simulink library "bcm"  (R2021b)
settings: Solver=VariableStepAuto  StartTime=0.0  StopTime=10.0  RelTol=1e-3
undefined symbols (not defined in the file or in its folder): KBCM_ShowUPT_cnt
libraries: simulink x33
(part 1 of 2)
settings Model: Creator=user  LastModifiedBy=FVT22063
settings SolverCC: AlgebraicLoopSolver=TrustRegion
settings DebuggingCC: SFMachineParentedDataDiag=warning

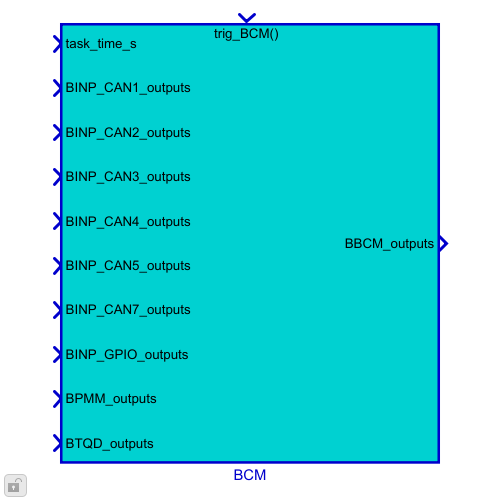
[thumbnail: Simulink's stored preview of the top-level diagram]
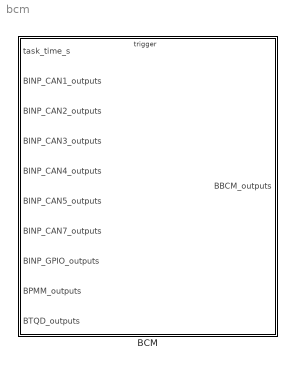
== system bcm ==
  BCM : Subsystem  TreatAsAtomicUnit=on
      settings: RTWSystemCode=Nonreusable function  RTWFcnNameOpts=Use subsystem name  RTWFileNameOpts=Use subsystem name

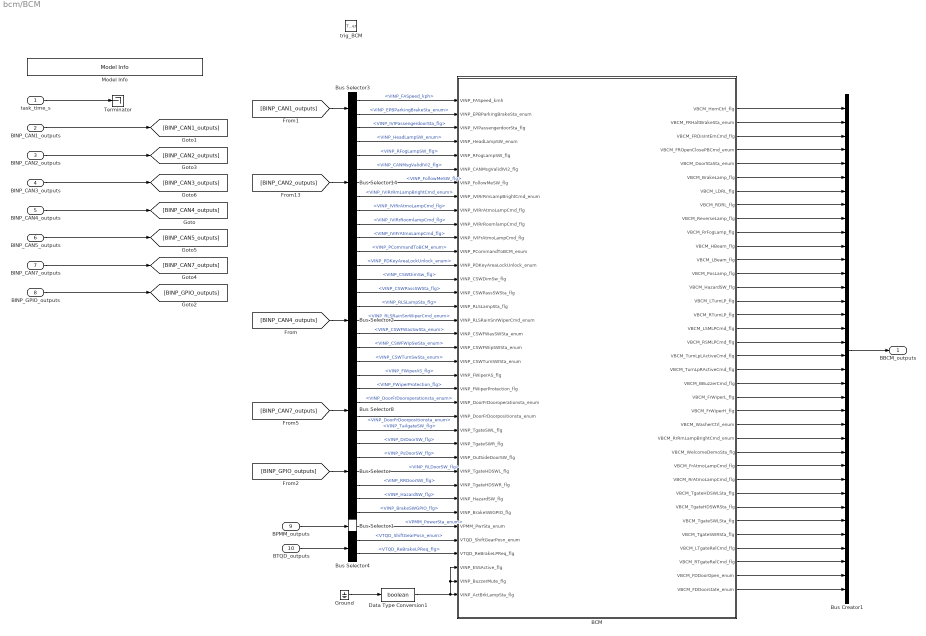
== system bcm/BCM ==
  task_time_s : Inport
  BINP_CAN1_outputs : Inport  Port=2  OutDataTypeStr=Bus: BINP_CAN1_outputs
  BINP_CAN2_outputs : Inport  Port=3  OutDataTypeStr=Bus: BINP_CAN2_outputs
  BINP_CAN3_outputs : Inport  Port=4  OutDataTypeStr=Bus: BINP_CAN3_outputs
  BINP_CAN4_outputs : Inport  Port=5  OutDataTypeStr=Bus: BINP_CAN4_outputs
  BINP_CAN5_outputs : Inport  Port=6  OutDataTypeStr=Bus: BINP_CAN5_outputs
  BINP_CAN7_outputs : Inport  Port=7  OutDataTypeStr=Bus: BINP_CAN7_outputs
  BINP_GPIO_outputs : Inport  Port=8  OutDataTypeStr=Bus: BINP_GPIO_outputs
  BPMM_outputs : Inport  Port=9  OutDataTypeStr=Bus: BPMM_outputs
  BTQD_outputs : Inport  Port=10  OutDataTypeStr=Bus: BTQD_outputs
  trig_BCM : TriggerPort  TriggerType=function-call  VariantControl=(inherit)
  BCM : Subsystem
  Bus Creator1 : BusCreator  Inputs=36  OutDataTypeStr=Bus: BBCM_outputs  NonVirtualBus=on
  Bus Selector : BusSelector  OutputSignals=VINP_TailgateSW_flg,VINP_DrDoorSW_flg,VINP_PsDoorSW_flg,VINP_RLDoorSW_flg,VINP_RRDoorSW_flg,VINP_HazardSW_flg,VINP_BrakeSWGPIO_flg
  Bus Selector1 : BusSelector  OutputSignals=VPMM_PowerSta_enum
  Bus Selector14 : BusSelector  OutputSignals=VINP_IVIPassengerdoorSta_flg,VINP_HeadLampSW_enum,VINP_RFogLampSW_flg,VINP_CANMsgValidIVI2_flg,VINP_FollowMeSW_flg,VINP_IVIRrRmLampBrightCmd_enum,VINP_IVIRrAtmoLampCmd_flg,VINP_IVIRrRoomlampCmd_flg,VINP_IVIFrAtmoLampCmd_flg
  Bus Selector2 : BusSelector  OutputSignals=VINP_PCommandToBCM_enum,VINP_PDKeyAreaLockUnlock_enum,VINP_CSWDimSw_flg,VINP_CSWPassSWSta_flg,VINP_RLSLampSta_flg,VINP_RLSRainSnrWiperCmd_enum,VINP_CSWFWasSwSta_enum,VINP_CSWFWipSwSta_enum,VINP_CSWTurnSwSta_enum,VINP_FWiperAS_flg,VINP_FWiperProtection_flg
  Bus Selector3 : BusSelector  OutputSignals=VINP_FASpeed_kph,VINP_EPBParkingBrakeSta_enum
  Bus Selector4 : BusSelector  OutputSignals=VTQD_ShiftGearPosn_enum,VTQD_ReBrakeLPReq_flg
  Bus Selector8 : BusSelector  OutputSignals=VINP_DoorFrDooroperationsta_enum,VINP_DoorFrDoorpositionsta_enum
  Data Type Conversion1 : DataTypeConversion  OutDataTypeStr=boolean
  Ground : Ground
  Model Info : simulink/Model-Wide Utilities/Model Info  Frame=on  DisplayStringWithTags=$Id: pmm.mdl 130 2021-02-08 12:40:01Z Shawn $  HorizontalTextAlignment=Center  LeftAlignmentValue=0.5
  Terminator : Terminator
  BBCM_outputs : Outport  OutDataTypeStr=Bus: BBCM_outputs  VectorParamsAs1DForOutWhenUnconnected=off
  wires:
  BPMM_outputs/1 -> Bus Selector1/1
  BINP_CAN4_outputs/1 -> [BINP_CAN4_outputs]
  BINP_CAN1_outputs/1 -> [BINP_CAN1_outputs]
  [BINP_CAN1_outputs] -> Bus Selector3/1
  BINP_GPIO_outputs/1 -> [BINP_GPIO_outputs]
  [BINP_GPIO_outputs] -> Bus Selector/1
  BINP_CAN2_outputs/1 -> [BINP_CAN2_outputs]
  BINP_CAN5_outputs/1 -> [BINP_CAN5_outputs]
  [BINP_CAN2_outputs] -> Bus Selector14/1
  BTQD_outputs/1 -> Bus Selector4/1
  [BINP_CAN4_outputs] -> Bus Selector2/1
  task_time_s/1 -> Terminator/1
  Bus Selector2/1 -> BCM/12(VINP_PCommandToBCM_enum)  "<VINP_PCommandToBCM_enum>"
  Bus Selector1/1 -> BCM/32(VPMM_PwrSta_enum)  "<VPMM_PowerSta_enum>"
  Bus Creator1/1 -> BBCM_outputs/1
  BINP_CAN3_outputs/1 -> [BINP_CAN3_outputs]
  Bus Selector3/1 -> BCM/1(VINP_FASpeed_kmh)  "<VINP_FASpeed_kph>"
  BCM/1(VBCM_HornCtrl_flg) -> Bus Creator1/1
  BCM/2(VBCM_FRHaltBrakeSta_enum) -> Bus Creator1/2
  BCM/3(VBCM_FRDisIntEmCmd_flg) -> Bus Creator1/3
  BCM/4(VBCM_FROpenClosePBCmd_enum) -> Bus Creator1/4
  BCM/5(VBCM_DoorStaSta_enum) -> Bus Creator1/5
  BCM/6(VBCM_BrakeLamp_flg) -> Bus Creator1/6
  BCM/7(VBCM_LDRL_flg) -> Bus Creator1/7
  BCM/8(VBCM_RDRL_flg) -> Bus Creator1/8
  BCM/9(VBCM_ReverseLamp_flg) -> Bus Creator1/9
  BCM/10(VBCM_RrFogLamp_flg) -> Bus Creator1/10
  BCM/11(VBCM_HBeam_flg) -> Bus Creator1/11
  BCM/12(VBCM_LBeam_flg) -> Bus Creator1/12
  BCM/13(VBCM_PosLamp_flg) -> Bus Creator1/13
  BCM/14(VBCM_HazardSW_flg) -> Bus Creator1/14
  BCM/15(VBCM_LTurnLP_flg) -> Bus Creator1/15
  BCM/16(VBCM_RTurnLP_flg) -> Bus Creator1/16
  BCM/17(VBCM_LSMLPCmd_flg) -> Bus Creator1/17
  BCM/18(VBCM_RSMLPCmd_flg) -> Bus Creator1/18
  BCM/19(VBCM_TurnLpLActiveCmd_flg) -> Bus Creator1/19
  BCM/20(VBCM_TurnLpRActiveCmd_flg) -> Bus Creator1/20
  BCM/21(VBCM_BBuzzerCmd_flg) -> Bus Creator1/21
  BCM/22(VBCM_FrWiperL_flg) -> Bus Creator1/22
  BCM/23(VBCM_FrWiperH_flg) -> Bus Creator1/23
  BCM/24(VBCM_WasherCtrl_enum) -> Bus Creator1/24
  BCM/25(VBCM_RrRmLampBrightCmd_enum) -> Bus Creator1/25
  BCM/26(VBCM_WelcomeDemoSta_flg) -> Bus Creator1/26
  BCM/27(VBCM_FrAtmoLampCmd_flg) -> Bus Creator1/27
  BCM/28(VBCM_RrAtmoLampCmd_flg) -> Bus Creator1/28
  BCM/29(VBCM_TgateHDSWLSta_flg) -> Bus Creator1/29
  BCM/30(VBCM_TgateHDSWRSta_flg) -> Bus Creator1/30
  BCM/31(VBCM_TgateSWLSta_flg) -> Bus Creator1/31
  BCM/32(VBCM_TgateSWRSta_flg) -> Bus Creator1/32
  BCM/33(VBCM_LTgateRelCmd_flg) -> Bus Creator1/33
  BCM/34(VBCM_RTgateRelCmd_flg) -> Bus Creator1/34
  BCM/35(VBCM_FDDoorOpen_enum) -> Bus Creator1/35
  BCM/36(VBCM_FDDoorstate_enum) -> Bus Creator1/36
  Bus Selector2/2 -> BCM/13(VINP_PDKeyAreaLockUnlock_enum)  "<VINP_PDKeyAreaLockUnlock_enum>"
  Bus Selector3/2 -> BCM/2(VINP_EPBParkingBrakeSta_enum)  "<VINP_EPBParkingBrakeSta_enum>"
  Bus Selector14/1 -> BCM/3(VINP_IVIPassengerdoorSta_flg)  "<VINP_IVIPassengerdoorSta_flg>"
  Bus Selector4/1 -> BCM/33(VTQD_ShiftGearPosn_enum)  "<VTQD_ShiftGearPosn_enum>"
  Bus Selector4/2 -> BCM/34(VTQD_ReBrakeLPReq_flg)  "<VTQD_ReBrakeLPReq_flg>"
  Bus Selector14/2 -> BCM/4(VINP_HeadLampSW_enum)  "<VINP_HeadLampSW_enum>"
  Bus Selector14/3 -> BCM/5(VINP_RFogLampSW_flg)  "<VINP_RFogLampSW_flg>"
  Bus Selector14/4 -> BCM/6(VINP_CANMsgValidIVI2_flg)  "<VINP_CANMsgValidIVI2_flg>"
  Bus Selector14/5 -> BCM/7(VINP_FollowMeSW_flg)  "<VINP_FollowMeSW_flg>"
  Bus Selector14/6 -> BCM/8(VINP_IVIRrRmLampBrightCmd_enum)  "<VINP_IVIRrRmLampBrightCmd_enum>"
  Bus Selector14/7 -> BCM/9(VINP_IVIRrAtmoLampCmd_flg)  "<VINP_IVIRrAtmoLampCmd_flg>"
  Bus Selector14/8 -> BCM/10(VINP_IVIRrRoomlampCmd_flg)  "<VINP_IVIRrRoomlampCmd_flg>"
  Bus Selector14/9 -> BCM/11(VINP_IVIFrAtmoLampCmd_flg)  "<VINP_IVIFrAtmoLampCmd_flg>"
  Bus Selector2/3 -> BCM/14(VINP_CSWDimSw_flg)  "<VINP_CSWDimSw_flg>"
  Bus Selector2/4 -> BCM/15(VINP_CSWPassSWSta_flg)  "<VINP_CSWPassSWSta_flg>"
  Bus Selector2/5 -> BCM/16(VINP_RLSLampSta_flg)  "<VINP_RLSLampSta_flg>"
  Bus Selector2/6 -> BCM/17(VINP_RLSRainSnrWiperCmd_enum)  "<VINP_RLSRainSnrWiperCmd_enum>"
  Bus Selector2/7 -> BCM/18(VINP_CSWFWasSWSta_enum)  "<VINP_CSWFWasSwSta_enum>"
  Bus Selector2/8 -> BCM/19(VINP_CSWFWipSWSta_enum)  "<VINP_CSWFWipSwSta_enum>"
  Bus Selector2/9 -> BCM/20(VINP_CSWTurnSWSta_enum)  "<VINP_CSWTurnSwSta_enum>"
  Data Type Conversion1/1 -> BCM/35(VINP_ESSActive_flg), BCM/36(VINP_BuzzerMute_flg), BCM/37(VINP_ActBrkLampSta_flg)
  Bus Selector2/10 -> BCM/21(VINP_FWiperAS_flg)  "<VINP_FWiperAS_flg>"
  Bus Selector2/11 -> BCM/22(VINP_FWiperProtection_flg)  "<VINP_FWiperProtection_flg>"
  BINP_CAN7_outputs/1 -> [BINP_CAN7_outputs]
  [BINP_CAN7_outputs] -> Bus Selector8/1
  Bus Selector8/1 -> BCM/23(VINP_DoorFrDooroperationsta_enum)  "<VINP_DoorFrDooroperationsta_enum>"
  Bus Selector8/2 -> BCM/24(VINP_DoorFrDoorpositionsta_enum)  "<VINP_DoorFrDoorpositionsta_enum>"
  Ground/1 -> Data Type Conversion1/1
  Bus Selector/3 -> BCM/27(VINP_OutSideDoorSW_flg)  "<VINP_PsDoorSW_flg>"
  Bus Selector/1 -> BCM/25(VINP_TgateSWL_flg)  "<VINP_TailgateSW_flg>"
  Bus Selector/4 -> BCM/28(VINP_TgateHDSWL_flg)  "<VINP_RLDoorSW_flg>"
  Bus Selector/5 -> BCM/29(VINP_TgateHDSWR_flg)  "<VINP_RRDoorSW_flg>"
  Bus Selector/7 -> BCM/31(VINP_BrakeSWGPIO_flg)  "<VINP_BrakeSWGPIO_flg>"
  Bus Selector/6 -> BCM/30(VINP_HazardSW_flg)  "<VINP_HazardSW_flg>"
  Bus Selector/2 -> BCM/26(VINP_TgateSWR_flg)  "<VINP_DrDoorSW_flg>"

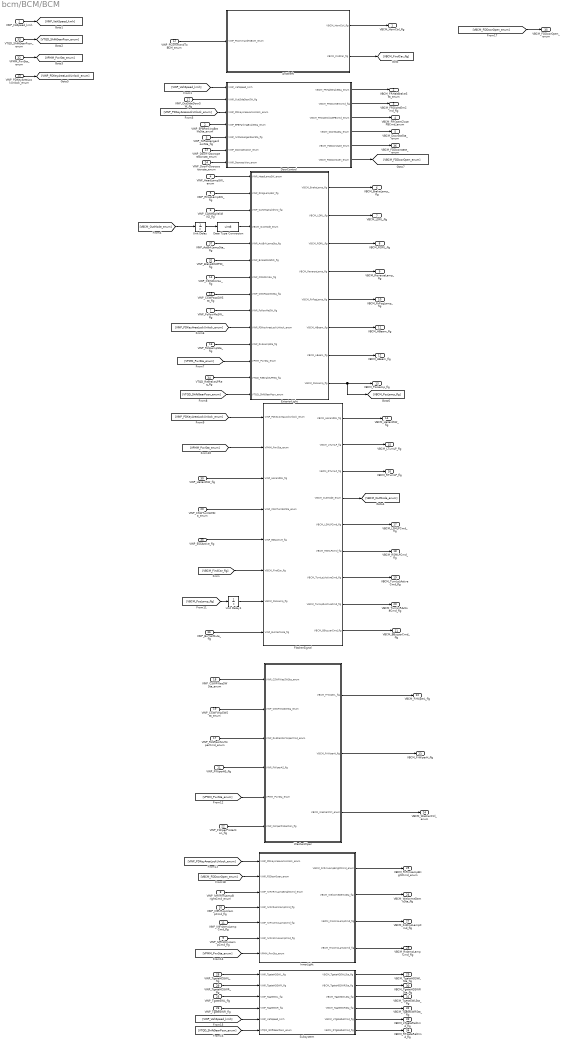
== system bcm/BCM/BCM ==
  VINP_FASpeed_kmh : Inport
  VINP_EPBParkingBrakeSta_enum : Inport  Port=2
  VINP_IVIPassengerdoorSta_flg : Inport  Port=3
  VINP_HeadLampSW_enum : Inport  Port=4
  VINP_RFogLampSW_flg : Inport  Port=5
  VINP_CANMsgValidIVI2_flg : Inport  Port=6
  VINP_FollowMeSW_flg : Inport  Port=7
  VINP_IVIRrRmLampBrightCmd_enum : Inport  Port=8
  VINP_IVIRrAtmoLampCmd_flg : Inport  Port=9
  VINP_IVIRrRoomlampCmd_flg : Inport  Port=10
  VINP_IVIFrAtmoLampCmd_flg : Inport  Port=11
  VINP_PCommandToBCM_enum : Inport  Port=12
  VINP_PDKeyAreaLockUnlock_enum : Inport  Port=13
  VINP_CSWDimSw_flg : Inport  Port=14
  VINP_CSWPassSWSta_flg : Inport  Port=15
  VINP_RLSLampSta_flg : Inport  Port=16
  VINP_RLSRainSnrWiperCmd_enum : Inport  Port=17
  VINP_CSWFWasSWSta_enum : Inport  Port=18
  VINP_CSWFWipSWSta_enum : Inport  Port=19
  VINP_CSWTurnSWSta_enum : Inport  Port=20
  VINP_FWiperAS_flg : Inport  Port=21
  VINP_FWiperProtection_flg : Inport  Port=22
  VINP_DoorFrDooroperationsta_enum : Inport  Port=23
  VINP_DoorFrDoorpositionsta_enum : Inport  Port=24
  VINP_TgateSWL_flg : Inport  Port=25
  VINP_TgateSWR_flg : Inport  Port=26
  VINP_OutSideDoorSW_flg : Inport  Port=27
  VINP_TgateHDSWL_flg : Inport  Port=28
  VINP_TgateHDSWR_flg : Inport  Port=29
  VINP_HazardSW_flg : Inport  Port=30
  VINP_BrakeSWGPIO_flg : Inport  Port=31
  VPMM_PwrSta_enum : Inport  Port=32
  VTQD_ShiftGearPosn_enum : Inport  Port=33
  VTQD_ReBrakeLPReq_flg : Inport  Port=34
  VINP_ESSActive_flg : Inport  Port=35
  VINP_BuzzerMute_flg : Inport  Port=36
  VINP_ActBrkLampSta_flg : Inport  Port=37
  Antitheft : Subsystem
  Data Type Conversion : DataTypeConversion  OutDataTypeStr=uint8
  DoorControl : Subsystem
  ExteriorLight : Subsystem
  FlasherSignal : Subsystem
  InnerLight : Subsystem
  Subsystem : Subsystem
  Unit Delay : UnitDelay  SampleTime=-1  HasFrameUpgradeWarning=on
  Unit Delay1 : UnitDelay  SampleTime=-1  HasFrameUpgradeWarning=on
  WasherWiper : Subsystem
  VBCM_HornCtrl_flg : Outport
  VBCM_FRHaltBrakeSta_enum : Outport  Port=2
  VBCM_FRDisIntEmCmd_flg : Outport  Port=3
  VBCM_FROpenClosePBCmd_enum : Outport  Port=4
  VBCM_DoorStaSta_enum : Outport  Port=5
  VBCM_BrakeLamp_flg : Outport  Port=6
  VBCM_LDRL_flg : Outport  Port=7
  VBCM_RDRL_flg : Outport  Port=8
  VBCM_ReverseLamp_flg : Outport  Port=9
  VBCM_RrFogLamp_flg : Outport  Port=10
  VBCM_HBeam_flg : Outport  Port=11
  VBCM_LBeam_flg : Outport  Port=12
  VBCM_PosLamp_flg : Outport  Port=13
  VBCM_HazardSW_flg : Outport  Port=14
  VBCM_LTurnLP_flg : Outport  Port=15
  VBCM_RTurnLP_flg : Outport  Port=16
  VBCM_LSMLPCmd_flg : Outport  Port=17
  VBCM_RSMLPCmd_flg : Outport  Port=18
  VBCM_TurnLpLActiveCmd_flg : Outport  Port=19
  VBCM_TurnLpRActiveCmd_flg : Outport  Port=20
  VBCM_BBuzzerCmd_flg : Outport  Port=21
  VBCM_FrWiperL_flg : Outport  Port=22
  VBCM_FrWiperH_flg : Outport  Port=23
  VBCM_WasherCtrl_enum : Outport  Port=24
  VBCM_RrRmLampBrightCmd_enum : Outport  Port=25
  VBCM_WelcomeDemoSta_flg : Outport  Port=26
  VBCM_FrAtmoLampCmd_flg : Outport  Port=27
  VBCM_RrAtmoLampCmd_flg : Outport  Port=28
  VBCM_TgateHDSWLSta_flg : Outport  Port=29
  VBCM_TgateHDSWRSta_flg : Outport  Port=30
  VBCM_TgateSWLSta_flg : Outport  Port=31
  VBCM_TgateSWRSta_flg : Outport  Port=32
  VBCM_LTgateRelCmd_flg : Outport  Port=33
  VBCM_RTgateRelCmd_flg : Outport  Port=34
  VBCM_FDDoorOpen_enum : Outport  Port=35
  VBCM_FDDoorstate_enum : Outport  Port=36
  wires:
  FlasherSignal/6(VBCM_RSMLPCmd_flg) -> VBCM_RSMLPCmd_flg/1
  VINP_ActBrkLampSta_flg/1 -> ExteriorLight/5(VINP_ActBrkLampSta_flg)
  VINP_IVIRrAtmoLampCmd_flg/1 -> InnerLight/6(VINP_IVIRrAtmoLampCmd_flg)
  VINP_TgateSWR_flg/1 -> Subsystem/4(VINP_TgateSWR_flg)
  VINP_TgateHDSWR_flg/1 -> Subsystem/2(VINP_TgateHDSWR_flg)
  VINP_ESSActive_flg/1 -> FlasherSignal/5(VINP_ESSActive_flg)
  VINP_TgateHDSWL_flg/1 -> Subsystem/1(VINP_TgateHDSWL_flg)
  FlasherSignal/5(VBCM_LSMLPCmd_flg) -> VBCM_LSMLPCmd_flg/1
  VINP_IVIRrRoomlampCmd_flg/1 -> InnerLight/4(VINP_IVIRrRoomlampCmd_flg)
  VINP_IVIFrAtmoLampCmd_flg/1 -> InnerLight/5(VINP_IVIFrAtmoLampCmd_flg)
  FlasherSignal/4(VBCM_OutMode_enum) -> [VBCM_OutMode_enum]
  VINP_IVIRrRmLampBrightCmd_enum/1 -> InnerLight/3(VINP_IVIRrRmLampBrightCmd_enum)
  [VINP_VehSpeed_kmh] -> Subsystem/5(VINP_VehSpeed_kmh)
  VINP_HeadLampSW_enum/1 -> ExteriorLight/1(VINP_HeadLampSW_enum)
  [VINP_PDKeyAreaLockUnlock_enum] -> FlasherSignal/1(VINP_PDKeyAreaLockUnlock_enum)
  VINP_FWiperAS_flg/1 -> WasherWiper/4(VINP_FWiperAS_flg)
  [VPMM_PwrSta_enum] -> ExteriorLight/12(VPMM_PwrSta_enum)
  Unit Delay1/1 -> FlasherSignal/7(VBCM_PosLamp_flg)
  [VINP_PDKeyAreaLockUnlock_enum] -> DoorControl/3(VINP_PDKeyAreaLockUnlock_enum)
  DoorControl/1(VBCM_FRHaltBrakeSta_enum) -> VBCM_FRHaltBrakeSta_enum/1
  VINP_RLSRainSnrWiperCmd_enum/1 -> WasherWiper/3(VINP_RLSRainSnrWiperCmd_enum)
  VINP_CSWFWipSWSta_enum/1 -> WasherWiper/2(VINP_CSWFWipSWSta_enum)
  [VBCM_PosLamp_flg] -> Unit Delay1/1
  VINP_BuzzerMute_flg/1 -> FlasherSignal/8(VINP_BuzzerMute_flg)
  VINP_FWiperProtection_flg/1 -> WasherWiper/6(VINP_FWiperProtection_flg)
  [VINP_PDKeyAreaLockUnlock_enum] -> InnerLight/1(VINP_PDKeyAreaLockUnlock_enum)
  VINP_CSWFWasSWSta_enum/1 -> WasherWiper/1(VINP_CSWFWasSWSta_enum)
  VINP_BrakeSWGPIO_flg/1 -> ExteriorLight/6(VINP_BrakeSWGPIO_flg)
  ExteriorLight/4(VBCM_ReverseLamp_flg) -> VBCM_ReverseLamp_flg/1
  [VPMM_PwrSta_enum] -> WasherWiper/5(VPMM_PwrSta_enum)
  VINP_CSWTurnSWSta_enum/1 -> FlasherSignal/4(VINP_CSWTurnSWSta_enum)
  [VINP_PDKeyAreaLockUnlock_enum] -> ExteriorLight/10(VINP_PDKeyAreaLockUnlock_enum)
  VINP_HazardSW_flg/1 -> FlasherSignal/3(VINP_HazardSW_flg)
  VINP_CANMsgValidIVI2_flg/1 -> ExteriorLight/3(VINP_CANMsgValidIVI2_flg)
  VINP_CSWDimSw_flg/1 -> ExteriorLight/7(VINP_CSWDimSw_flg)
  [VTQD_ShiftGearPosn_enum] -> ExteriorLight/14(VTQD_ShiftGearPosn_enum)
  ExteriorLight/2(VBCM_LDRL_flg) -> VBCM_LDRL_flg/1
  VINP_RLSLampSta_flg/1 -> ExteriorLight/11(VINP_RLSLampSta_flg)
  VINP_CSWPassSWSta_flg/1 -> ExteriorLight/8(VINP_CSWPassSWSta_flg)
  VINP_PDKeyAreaLockUnlock_enum/1 -> [VINP_PDKeyAreaLockUnlock_enum]
  VINP_RFogLampSW_flg/1 -> ExteriorLight/2(VINP_RFogLampSW_flg)
  VINP_EPBParkingBrakeSta_enum/1 -> DoorControl/4(VINP_EPBParkingBrakeSta_enum)
  VINP_FASpeed_kmh/1 -> [VINP_VehSpeed_kmh]
  DoorControl/4(VBCM_DoorStaSta_enum) -> VBCM_DoorStaSta_enum/1
  Unit Delay/1 -> Data Type Conversion/1
  Antitheft/2(VBCM_FindCar_flg) -> [VBCM_FindCar_flg]
  [VBCM_FindCar_flg] -> FlasherSignal/6(VBCM_FindCar_flg)
  Antitheft/1(VBCM_HornCtrl_flg) -> VBCM_HornCtrl_flg/1
  InnerLight/4(VBCM_RrAtmoLampCmd_flg) -> VBCM_RrAtmoLampCmd_flg/1
  FlasherSignal/9(VBCM_BBuzzerCmd_flg) -> VBCM_BBuzzerCmd_flg/1
  InnerLight/2(VBCM_WelcomeDemoSta_flg) -> VBCM_WelcomeDemoSta_flg/1
  [VBCM_OutMode_enum] -> Unit Delay/1
  ExteriorLight/3(VBCM_RDRL_flg) -> VBCM_RDRL_flg/1
  FlasherSignal/3(VBCM_RTurnLP_flg) -> VBCM_RTurnLP_flg/1
  WasherWiper/1(VBCM_FrWiperL_flg) -> VBCM_FrWiperL_flg/1
  VINP_PCommandToBCM_enum/1 -> Antitheft/1(VINP_PCommandToBCM_enum)
  VINP_TgateSWL_flg/1 -> Subsystem/3(VINP_TgateSWL_flg)
  ExteriorLight/5(VBCM_RrFogLamp_flg) -> VBCM_RrFogLamp_flg/1
  InnerLight/3(VBCM_FrAtmoLampCmd_flg) -> VBCM_FrAtmoLampCmd_flg/1
  InnerLight/1(VBCM_RrRmLampBrightCmd_enum) -> VBCM_RrRmLampBrightCmd_enum/1
  DoorControl/2(VBCM_FRDisIntEmCmd_flg) -> VBCM_FRDisIntEmCmd_flg/1
  VPMM_PwrSta_enum/1 -> [VPMM_PwrSta_enum]
  VINP_FollowMeSW_flg/1 -> ExteriorLight/9(VINP_FollowMeSW_flg)
  VINP_IVIPassengerdoorSta_flg/1 -> DoorControl/5(VINP_IVIPassengerdoorSta_flg)
  WasherWiper/2(VBCM_FrWiperH_flg) -> VBCM_FrWiperH_flg/1
  ExteriorLight/8(VBCM_PosLamp_flg) -> [VBCM_PosLamp_flg], VBCM_PosLamp_flg/1
  [VBCM_FDDoorOpen_enum] -> VBCM_FDDoorOpen_enum/1
  DoorControl/6(VBCM_FDDoorOpen_enum) -> [VBCM_FDDoorOpen_enum]
  Subsystem/6(VBCM_RTgateRelCmd_flg) -> VBCM_RTgateRelCmd_flg/1
  Subsystem/1(VBCM_TgateHDSWLSta_flg) -> VBCM_TgateHDSWLSta_flg/1
  VINP_OutSideDoorSW_flg/1 -> DoorControl/2(VINP_OutSideDoorSW_flg)
  Subsystem/2(VBCM_TgateHDSWRSta_flg) -> VBCM_TgateHDSWRSta_flg/1
  [VPMM_PwrSta_enum] -> FlasherSignal/2(VPMM_PwrSta_enum)
  VTQD_ReBrakeLPReq_flg/1 -> ExteriorLight/13(VTQD_ReBrakeLPReq_flg)
  VTQD_ShiftGearPosn_enum/1 -> [VTQD_ShiftGearPosn_enum]
  Subsystem/4(VBCM_TgateSWRSta_flg) -> VBCM_TgateSWRSta_flg/1
  WasherWiper/3(VBCM_WasherCtrl_enum) -> VBCM_WasherCtrl_enum/1
  DoorControl/3(VBCM_FROpenClosePBCmd_enum) -> VBCM_FROpenClosePBCmd_enum/1
  Subsystem/5(VBCM_LTgateRelCmd_flg) -> VBCM_LTgateRelCmd_flg/1
  [VBCM_FDDoorOpen_enum] -> InnerLight/2(VINP_FDDoorOpen_enum)
  FlasherSignal/8(VBCM_TurnLpRActiveCmd_flg) -> VBCM_TurnLpRActiveCmd_flg/1
  ExteriorLight/1(VBCM_BrakeLamp_flg) -> VBCM_BrakeLamp_flg/1
  [VPMM_PwrSta_enum] -> InnerLight/7(VPMM_PwrSta_enum)
  Subsystem/3(VBCM_TgateSWLSta_flg) -> VBCM_TgateSWLSta_flg/1
  FlasherSignal/7(VBCM_TurnLpLActiveCmd_flg) -> VBCM_TurnLpLActiveCmd_flg/1
  [VTQD_ShiftGearPosn_enum] -> Subsystem/6(VTQD_ShiftGearPosn_enum)
  ExteriorLight/6(VBCM_HBeam_flg) -> VBCM_HBeam_flg/1
  [VINP_VehSpeed_kmh] -> DoorControl/1(VINP_VehSpeed_kmh)
  FlasherSignal/2(VBCM_LTurnLP_flg) -> VBCM_LTurnLP_flg/1
  FlasherSignal/1(VBCM_HazardSW_flg) -> VBCM_HazardSW_flg/1
  ExteriorLight/7(VBCM_LBeam_flg) -> VBCM_LBeam_flg/1
  VINP_DoorFrDooroperationsta_enum/1 -> DoorControl/6(VINP_Dooroperation_enum)
  VINP_DoorFrDoorpositionsta_enum/1 -> DoorControl/7(VINP_Doorposition_enum)
  DoorControl/5(VBCM_FDDoorstate_enum) -> VBCM_FDDoorstate_enum/1
  Data Type Conversion/1 -> ExteriorLight/4(VBCM_OutMode_enum)

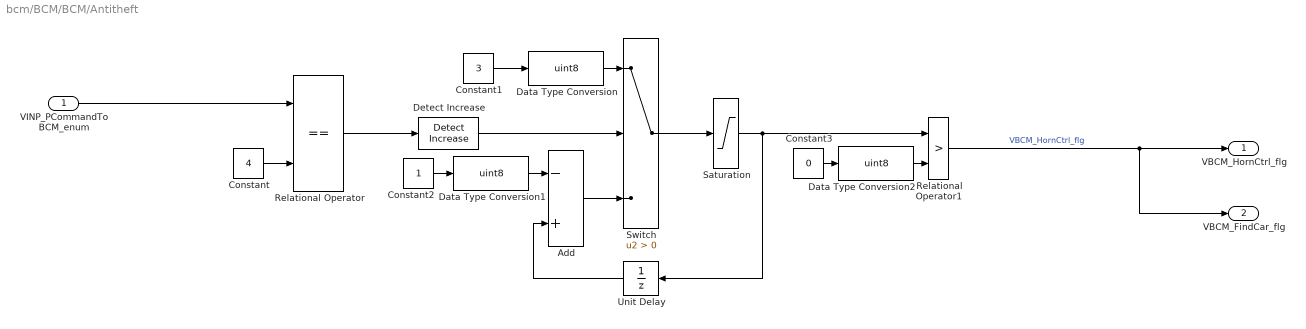
== system bcm/BCM/BCM/Antitheft ==
  VINP_PCommandToBCM_enum : Inport
  Add : Sum  Inputs=-+
  Constant : Constant  Value=4
  Constant1 : Constant  Value=3
  Constant2 : Constant
  Constant3 : Constant  Value=0
  Data Type Conversion : DataTypeConversion  OutDataTypeStr=uint8
  Data Type Conversion1 : DataTypeConversion  OutDataTypeStr=uint8
  Data Type Conversion2 : DataTypeConversion  OutDataTypeStr=uint8
  Detect Increase : simulink/Logic and Bit Operations/Detect Increase  vinit=0.0  OutDataTypeStr=boolean
  Relational Operator : RelationalOperator  Operator===  OutDataTypeStr=boolean  RndMeth=Simplest
  Relational Operator1 : RelationalOperator  Operator=>  OutDataTypeStr=boolean  RndMeth=Simplest
  Saturation : Saturate  UpperLimit=3  LowerLimit=0
  Switch : Switch  Criteria=u2 > Threshold
  Unit Delay : UnitDelay  SampleTime=-1  HasFrameUpgradeWarning=on
  VBCM_HornCtrl_flg : Outport
  VBCM_FindCar_flg : Outport  Port=2
  wires:
  Relational Operator1/1 -> VBCM_FindCar_flg/1, VBCM_HornCtrl_flg/1  "VBCM_HornCtrl_flg"
  Constant2/1 -> Data Type Conversion1/1
  Data Type Conversion1/1 -> Add/1
  Saturation/1 -> Unit Delay/1, Relational Operator1/1
  Detect Increase/1 -> Switch/2
  VINP_PCommandToBCM_enum/1 -> Relational Operator/1
  Data Type Conversion/1 -> Switch/1
  Switch/1 -> Saturation/1
  Constant1/1 -> Data Type Conversion/1
  Data Type Conversion2/1 -> Relational Operator1/2
  Constant/1 -> Relational Operator/2
  Constant3/1 -> Data Type Conversion2/1
  Relational Operator/1 -> Detect Increase/1
  Unit Delay/1 -> Add/2
  Add/1 -> Switch/3

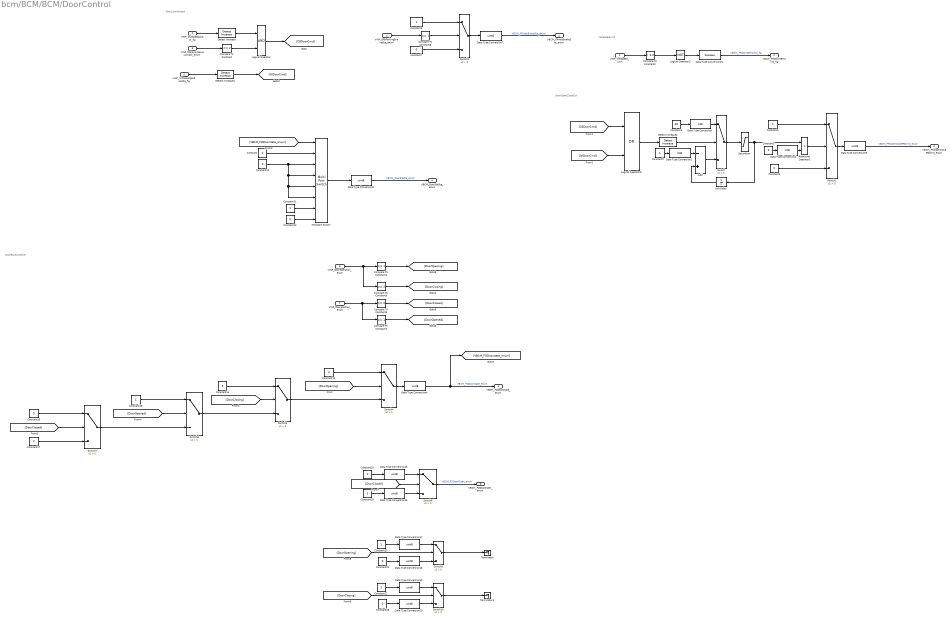
== system bcm/BCM/BCM/DoorControl ==
  note: DoorECUtoVehcle
  note: VehSpeedLimit
  note: DoorOpenCloseCtrl
  note: DoorControlInput
  VINP_VehSpeed_kmh : Inport
  VINP_OutSideDoorSW_flg : Inport  Port=2
  VINP_PDKeyAreaLockUnlock_enum : Inport  Port=3
  VINP_EPBParkingBrakeSta_enum : Inport  Port=4
  VINP_IVIPassengerdoorSta_flg : Inport  Port=5
  VINP_Dooroperation_enum : Inport  Port=6
  VINP_Doorposition_enum : Inport  Port=7
  Add : Sum  Inputs=-+
  Compare To Constant : simulink/Logic and Bit Operations/Compare To Constant  relop===  const=2  OutDataTypeStr=boolean
  Compare To Constant2 : simulink/Logic and Bit Operations/Compare To Constant  relop=>  const=3.0  OutDataTypeStr=boolean
  Compare To Constant3 : simulink/Logic and Bit Operations/Compare To Constant  relop===  const=1  OutDataTypeStr=boolean
  Compare To Constant4 : simulink/Logic and Bit Operations/Compare To Constant  relop===  const=1  OutDataTypeStr=boolean
  Compare To Constant5 : simulink/Logic and Bit Operations/Compare To Constant  relop===  const=2  OutDataTypeStr=boolean
  Compare To Constant6 : simulink/Logic and Bit Operations/Compare To Constant  relop===  const=0  OutDataTypeStr=boolean
  Compare To Constant7 : simulink/Logic and Bit Operations/Compare To Constant  relop===  const=1  OutDataTypeStr=boolean
  Constant : Constant  Value=2
  Constant1 : Constant  Value=30
  Constant{3,5,7,10,16,18,21,23} (8 alike) : Constant  Value=0
  Constant{2,4,6,11,15,19..20,22} (8 alike) : Constant
  Constant12 : Constant  Value=2
  Constant13 : Constant  Value=4
  Constant14 : Constant  Value=5
  Constant17 : Constant  Value=2
  Data Type Conversion : DataTypeConversion  OutDataTypeStr=int8
  Data Type Conversion1 : DataTypeConversion  OutDataTypeStr=int8
  Data Type Conversion{4..5,7,9,15..20} (10 alike) : DataTypeConversion  OutDataTypeStr=uint8
  Data Type Conversion2 : DataTypeConversion  OutDataTypeStr=int8
  Data Type Conversion21 : DataTypeConversion  OutDataTypeStr=boolean
  Detect Increase : simulink/Logic and Bit Operations/Detect Increase  vinit=0.0  OutDataTypeStr=boolean
  Detect Increase1 : simulink/Logic and Bit Operations/Detect Increase  vinit=0.0  OutDataTypeStr=boolean
  Detect Increase2 : simulink/Logic and Bit Operations/Detect Increase  vinit=0.0  OutDataTypeStr=boolean
  Logical Operator : Logic  AllPortsSameDT=off  OutDataTypeStr=boolean
  Logical Operator2 : Logic  Operator=NOT  AllPortsSameDT=off  OutDataTypeStr=boolean
  Logical Operator3 : Logic  Operator=OR  AllPortsSameDT=off  OutDataTypeStr=boolean
  Multiport Switch : MultiPortSwitch  DataPortOrder=Zero-based contiguous  Inputs=7  DiagnosticForDefault=None  zeroidx=on
  Relational Operator1 : RelationalOperator  Operator=>  OutDataTypeStr=boolean  RndMeth=Simplest
  Saturation : Saturate  UpperLimit=30  LowerLimit=0
  Switch{,1..2,4..10} (10 alike) : Switch  Criteria=u2 > Threshold
  Terminator : Terminator
  Terminator1 : Terminator
  Unit Delay : UnitDelay  SampleTime=-1  HasFrameUpgradeWarning=on
  VBCM_FRHaltBrakeSta_enum : Outport
  VBCM_FRDisIntEmCmd_flg : Outport  Port=2
  VBCM_FROpenClosePBCmd_enum : Outport  Port=3
  VBCM_DoorStaSta_enum : Outport  Port=4
  VBCM_FDDoorstate_enum : Outport  Port=5
  VBCM_FDDoorOpen_enum : Outport  Port=6
  wires:
  VINP_OutSideDoorSW_flg/1 -> Detect Increase/1
  VINP_PDKeyAreaLockUnlock_enum/1 -> Compare To Constant/1
  Detect Increase/1 -> Logical Operator/1
  Compare To Constant/1 -> Logical Operator/2
  Logical Operator/1 -> [OSDoorCmd]
  VINP_IVIPassengerdoorSta_flg/1 -> Detect Increase1/1
  Detect Increase1/1 -> [IVIDoorCmd]
  VINP_VehSpeed_kmh/1 -> Compare To Constant2/1
  Compare To Constant2/1 -> Logical Operator2/1
  Logical Operator2/1 -> Data Type Conversion21/1
  [OSDoorCmd] -> Logical Operator3/1
  [IVIDoorCmd] -> Logical Operator3/2
  Add/1 -> Switch/3
  Logical Operator3/1 -> Detect Increase2/1
  Unit Delay/1 -> Add/2
  Constant3/1 -> Data Type Conversion2/1
  Data Type Conversion2/1 -> Relational Operator1/2
  Detect Increase2/1 -> Switch/2
  Constant2/1 -> Data Type Conversion1/1
  Saturation/1 -> Unit Delay/1, Relational Operator1/1
  Data Type Conversion1/1 -> Add/1
  Switch/1 -> Saturation/1
  Constant1/1 -> Data Type Conversion/1
  Data Type Conversion/1 -> Switch/1
  Switch1/1 -> Data Type Conversion5/1
  Relational Operator1/1 -> Switch1/2
  Constant4/1 -> Switch1/1
  VINP_EPBParkingBrakeSta_enum/1 -> Compare To Constant3/1
  Compare To Constant3/1 -> Switch2/2
  Switch2/1 -> Data Type Conversion7/1
  Constant6/1 -> Switch2/1
  Constant7/1 -> Switch2/3
  Constant/1 -> Multiport Switch/2
  Multiport Switch/1 -> Data Type Conversion9/1
  Constant10/1 -> Multiport Switch/6, Multiport Switch/5, Multiport Switch/4, Multiport Switch/3
  Constant11/1 -> Multiport Switch/7
  Data Type Conversion9/1 -> VBCM_DoorStaSta_enum/1  "VBCM_DoorStaSta_enum"
  Constant12/1 -> Multiport Switch/8
  VINP_Dooroperation_enum/1 -> Compare To Constant5/1, Compare To Constant4/1
  Compare To Constant4/1 -> [DoorOpening]
  Compare To Constant5/1 -> [DoorClosing]
  VINP_Doorposition_enum/1 -> Compare To Constant7/1, Compare To Constant6/1
  Compare To Constant6/1 -> [DoorClosed]
  Compare To Constant7/1 -> [DoorOpened]
  [DoorOpening] -> Switch4/2
  Constant13/1 -> Switch4/1
  Switch5/1 -> Switch4/3
  [DoorClosing] -> Switch5/2
  Constant14/1 -> Switch5/1
  Switch6/1 -> Switch5/3
  [DoorOpened] -> Switch6/2
  Constant15/1 -> Switch6/1
  Constant16/1 -> Switch7/1
  [DoorClosed] -> Switch7/2
  Switch7/1 -> Switch6/3
  Constant17/1 -> Switch7/3
  Switch4/1 -> Data Type Conversion4/1
  [VBCM_FDDoorstate_enum] -> Multiport Switch/1
  [DoorClosed] -> Switch8/2
  Constant18/1 -> Data Type Conversion15/1
  Data Type Conversion15/1 -> Switch8/1
  Constant19/1 -> Data Type Conversion16/1
  Data Type Conversion16/1 -> Switch8/3
  Switch8/1 -> VBCM_FDDoorOpen_enum/1  "VBCM_FDDoorOpen_enum"
  [DoorOpening] -> Switch9/2
  Data Type Conversion17/1 -> Switch9/1
  Constant20/1 -> Data Type Conversion17/1
  Data Type Conversion18/1 -> Switch9/3
  Constant21/1 -> Data Type Conversion18/1
  Switch9/1 -> Terminator/1
  Switch10/1 -> Terminator1/1
  Constant23/1 -> Data Type Conversion20/1
  Data Type Conversion20/1 -> Switch10/3
  Constant22/1 -> Data Type Conversion19/1
  Data Type Conversion19/1 -> Switch10/1
  [DoorClosing] -> Switch10/2
  Data Type Conversion21/1 -> VBCM_FRDisIntEmCmd_flg/1  "VBCM_FRDisIntEmCmd_flg"
  Data Type Conversion7/1 -> VBCM_FRHaltBrakeSta_enum/1  "VBCM_FRHaltBrakeSta_enum"
  Data Type Conversion5/1 -> VBCM_FROpenClosePBCmd_enum/1  "VBCM_FROpenClosePBCmd_enum"
  Constant5/1 -> Switch1/3
  Data Type Conversion4/1 -> VBCM_FDDoorstate_enum/1, [VBCM_FDDoorstate_enum]  "VBCM_FDDoorstate_enum"

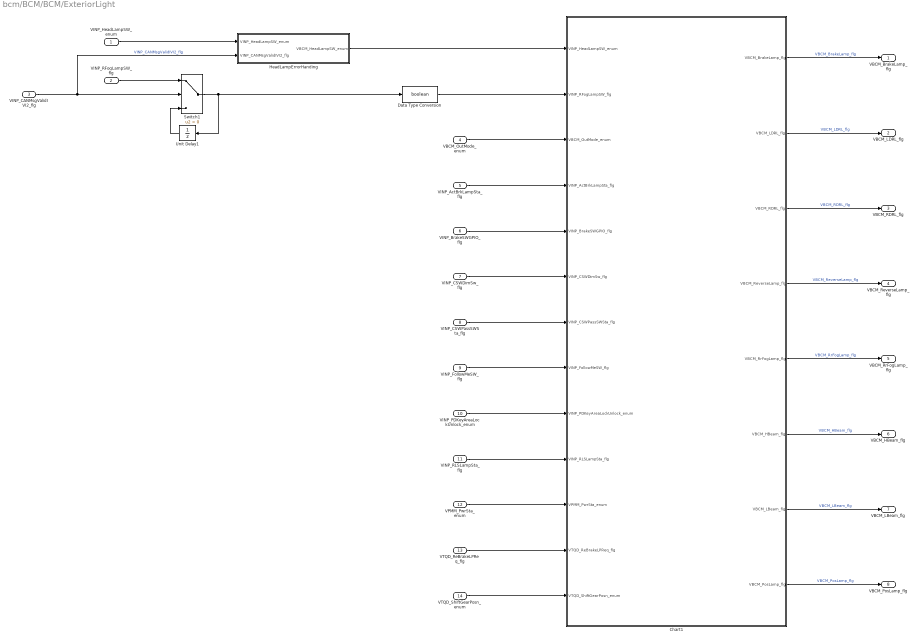
== system bcm/BCM/BCM/ExteriorLight ==
  VINP_HeadLampSW_enum : Inport
  VINP_RFogLampSW_flg : Inport  Port=2
  VINP_CANMsgValidIVI2_flg : Inport  Port=3
  VBCM_OutMode_enum : Inport  Port=4
  VINP_ActBrkLampSta_flg : Inport  Port=5
  VINP_BrakeSWGPIO_flg : Inport  Port=6
  VINP_CSWDimSw_flg : Inport  Port=7
  VINP_CSWPassSWSta_flg : Inport  Port=8
  VINP_FollowMeSW_flg : Inport  Port=9
  VINP_PDKeyAreaLockUnlock_enum : Inport  Port=10
  VINP_RLSLampSta_flg : Inport  Port=11
  VPMM_PwrSta_enum : Inport  Port=12
  VTQD_ReBrakeLPReq_flg : Inport  Port=13
  VTQD_ShiftGearPosn_enum : Inport  Port=14
  Chart1 : Stateflow chart  TreatAsAtomicUnit=on
      settings: PortSchema="{\"entries\":[{\"content\":{\"sides\":[{\"content\":{\"connectorIds\":[\"In7\",\"In9\",\"In1\",\"In2\",\"In3\",\"In4\",\"In5\",\"In6\",\"In8\",\"In10\",\"In11\",\"In12\",\"In13\"]},\"type\":\"ConnectorPlacement.EquallySpacedRectSide\",\"uuid\":\"6fe89a48-cc4a-4979-bb2b-3532d5785f4a\"},{\"content\":{\"connectorIds\":[\"Out1\",\"Out2\",\"Out3\",\"Out4\",\"Out5\",\"Out6\",\"Out7\",\"Out8\"],\"side\":\"RIGHT\"},\"type\":\"ConnectorPlacement.EquallySpacedRectSide\",\"uuid\":\"c6809bb6-7b4c-4551-88d6-a11895f633ce\"},{\"content\":{\"connectorIds\":[],\"side\":\"TOP\"},\"type\":\"ConnectorPlacement.EquallySpacedRectSide\",\"uuid\":\"ff1c91a2-870b-40c1-8124-5ae0e202aebd\"}]},\"type\":\"ConnectorPlacement.EquallySpacedConnector\",\"uuid\":\"2cfd3adb-65e9-4d0e-88de-6b09ee5e18e1\"}],\"packageUris\":[\"http://schema.mathworks.com/mf0/Connector/R2020b\"],\"version\":\"1.0\"}"
  Data Type Conversion : DataTypeConversion  OutDataTypeStr=boolean
  HeadLampErrorHanding : Subsystem
  Switch1 : Switch  Criteria=u2 > Threshold
  Unit Delay1 : UnitDelay  SampleTime=-1  HasFrameUpgradeWarning=on
  VBCM_BrakeLamp_flg : Outport
  VBCM_LDRL_flg : Outport  Port=2
  VBCM_RDRL_flg : Outport  Port=3
  VBCM_ReverseLamp_flg : Outport  Port=4
  VBCM_RrFogLamp_flg : Outport  Port=5
  VBCM_HBeam_flg : Outport  Port=6
  VBCM_LBeam_flg : Outport  Port=7
  VBCM_PosLamp_flg : Outport  Port=8
  wires:
  Unit Delay1/1 -> Switch1/3
  VINP_CANMsgValidIVI2_flg/1 -> Switch1/2, HeadLampErrorHanding/2(VINP_CANMsgValidIVI2_flg)  "VINP_CANMsgValidIVI2_flg"
  Switch1/1 -> Unit Delay1/1, Data Type Conversion/1
  VINP_RFogLampSW_flg/1 -> Switch1/1
  VINP_HeadLampSW_enum/1 -> HeadLampErrorHanding/1(VINP_HeadLampSW_enum)
  HeadLampErrorHanding/1(VBCM_HeadLampSW_enum) -> Chart1/7(VINP_HeadLampSW_enum)
  VBCM_OutMode_enum/1 -> Chart1/1(VBCM_OutMode_enum)
  VINP_ActBrkLampSta_flg/1 -> Chart1/2(VINP_ActBrkLampSta_flg)
  VINP_BrakeSWGPIO_flg/1 -> Chart1/3(VINP_BrakeSWGPIO_flg)
  VINP_CSWDimSw_flg/1 -> Chart1/4(VINP_CSWDimSw_flg)
  VINP_CSWPassSWSta_flg/1 -> Chart1/5(VINP_CSWPassSWSta_flg)
  VINP_FollowMeSW_flg/1 -> Chart1/6(VINP_FollowMeSW_flg)
  VINP_PDKeyAreaLockUnlock_enum/1 -> Chart1/8(VINP_PDKeyAreaLockUnlock_enum)
  VINP_RLSLampSta_flg/1 -> Chart1/10(VINP_RLSLampSta_flg)
  VPMM_PwrSta_enum/1 -> Chart1/11(VPMM_PwrSta_enum)
  VTQD_ReBrakeLPReq_flg/1 -> Chart1/12(VTQD_ReBrakeLPReq_flg)
  VTQD_ShiftGearPosn_enum/1 -> Chart1/13(VTQD_ShiftGearPosn_enum)
  Chart1/5(VBCM_RrFogLamp_flg) -> VBCM_RrFogLamp_flg/1  "VBCM_RrFogLamp_flg"
  Chart1/6(VBCM_HBeam_flg) -> VBCM_HBeam_flg/1  "VBCM_HBeam_flg"
  Chart1/7(VBCM_LBeam_flg) -> VBCM_LBeam_flg/1  "VBCM_LBeam_flg"
  Chart1/8(VBCM_PosLamp_flg) -> VBCM_PosLamp_flg/1  "VBCM_PosLamp_flg"
  Chart1/1(VBCM_BrakeLamp_flg) -> VBCM_BrakeLamp_flg/1  "VBCM_BrakeLamp_flg"
  Chart1/2(VBCM_LDRL_flg) -> VBCM_LDRL_flg/1  "VBCM_LDRL_flg"
  Chart1/3(VBCM_RDRL_flg) -> VBCM_RDRL_flg/1  "VBCM_RDRL_flg"
  Chart1/4(VBCM_ReverseLamp_flg) -> VBCM_ReverseLamp_flg/1  "VBCM_ReverseLamp_flg"
  Data Type Conversion/1 -> Chart1/9(VINP_RFogLampSW_flg)

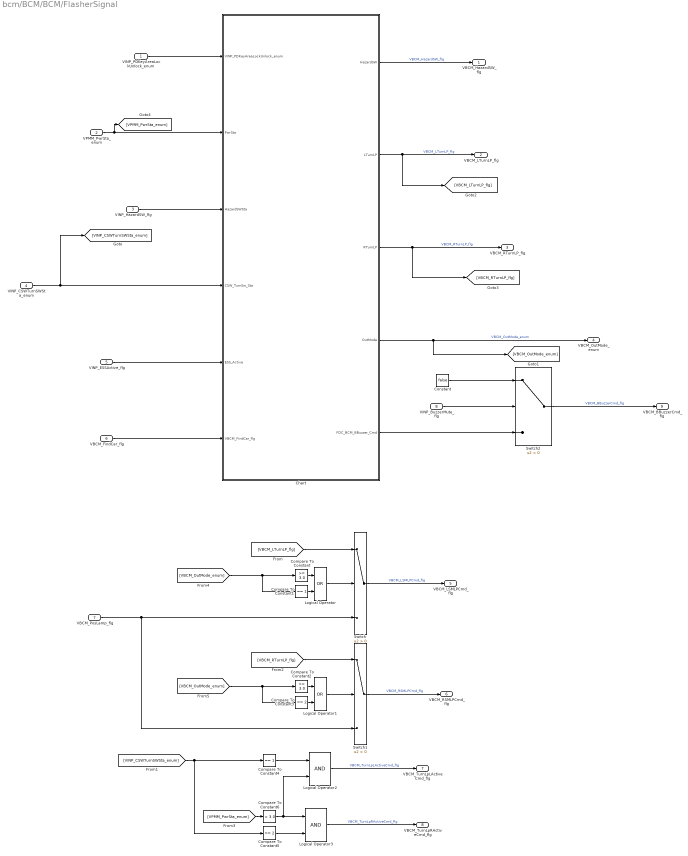
== system bcm/BCM/BCM/FlasherSignal ==
  VINP_PDKeyAreaLockUnlock_enum : Inport
  VPMM_PwrSta_enum : Inport  Port=2
  VINP_HazardSW_flg : Inport  Port=3
  VINP_CSWTurnSWSta_enum : Inport  Port=4
  VINP_ESSActive_flg : Inport  Port=5
  VBCM_FindCar_flg : Inport  Port=6
  VBCM_PosLamp_flg : Inport  Port=7
  VINP_BuzzerMute_flg : Inport  Port=8
  Chart : Stateflow chart  TreatAsAtomicUnit=on
  Compare To Constant : simulink/Logic and Bit Operations/Compare To Constant  relop=>=  const=3.0  OutDataTypeStr=boolean
  Compare To Constant1 : simulink/Logic and Bit Operations/Compare To Constant  relop===  const=1  OutDataTypeStr=boolean
  Compare To Constant2 : simulink/Logic and Bit Operations/Compare To Constant  relop=>=  const=3.0  OutDataTypeStr=boolean
  Compare To Constant3 : simulink/Logic and Bit Operations/Compare To Constant  relop===  const=2  OutDataTypeStr=boolean
  Compare To Constant4 : simulink/Logic and Bit Operations/Compare To Constant  relop===  const=1  OutDataTypeStr=boolean
  Compare To Constant5 : simulink/Logic and Bit Operations/Compare To Constant  relop===  const=2  OutDataTypeStr=boolean
  Compare To Constant6 : simulink/Logic and Bit Operations/Compare To Constant  relop=>  const=3.0  OutDataTypeStr=boolean
  Constant : Constant  Value=false
  Logical Operator : Logic  Operator=OR  AllPortsSameDT=off  OutDataTypeStr=boolean
  Logical Operator1 : Logic  Operator=OR  AllPortsSameDT=off  OutDataTypeStr=boolean
  Logical Operator2 : Logic  AllPortsSameDT=off  OutDataTypeStr=boolean
  Logical Operator3 : Logic  AllPortsSameDT=off  OutDataTypeStr=boolean
  Switch : Switch  Criteria=u2 > Threshold
  Switch1 : Switch  Criteria=u2 > Threshold
  Switch2 : Switch  Criteria=u2 > Threshold
  VBCM_HazardSW_flg : Outport
  VBCM_LTurnLP_flg : Outport  Port=2
  VBCM_RTurnLP_flg : Outport  Port=3
  VBCM_OutMode_enum : Outport  Port=4
  VBCM_LSMLPCmd_flg : Outport  Port=5
  VBCM_RSMLPCmd_flg : Outport  Port=6
  VBCM_TurnLpLActiveCmd_flg : Outport  Port=7
  VBCM_TurnLpRActiveCmd_flg : Outport  Port=8
  VBCM_BBuzzerCmd_flg : Outport  Port=9
  wires:
  Chart/1(HazardSW) -> VBCM_HazardSW_flg/1  "VBCM_HazardSW_flg"
  Chart/3(RTurnLP) -> [VBCM_RTurnLP_flg], VBCM_RTurnLP_flg/1  "VBCM_RTurnLP_flg"
  VINP_PDKeyAreaLockUnlock_enum/1 -> Chart/1(VINP_PDKeyAreaLockUnlock_enum)
  Chart/2(LTurnLP) -> [VBCM_LTurnLP_flg], VBCM_LTurnLP_flg/1  "VBCM_LTurnLP_flg"
  VPMM_PwrSta_enum/1 -> [VPMM_PwrSta_enum], Chart/2(PwrSta)
  VINP_HazardSW_flg/1 -> Chart/3(HazardSWSta)
  Chart/4(OutMode) -> [VBCM_OutMode_enum], VBCM_OutMode_enum/1  "VBCM_OutMode_enum"
  VINP_ESSActive_flg/1 -> Chart/5(ESS_Active)
  VBCM_FindCar_flg/1 -> Chart/6(VBCM_FindCar_flg)
  VBCM_PosLamp_flg/1 -> Switch1/3, Switch/3
  [VBCM_OutMode_enum] -> Compare To Constant1/1, Compare To Constant/1
  Logical Operator/1 -> Switch/2
  Compare To Constant/1 -> Logical Operator/1
  Compare To Constant1/1 -> Logical Operator/2
  [VBCM_LTurnLP_flg] -> Switch/1
  Switch/1 -> VBCM_LSMLPCmd_flg/1  "VBCM_LSMLPCmd_flg"
  Switch1/1 -> VBCM_RSMLPCmd_flg/1  "VBCM_RSMLPCmd_flg"
  [VBCM_RTurnLP_flg] -> Switch1/1
  Compare To Constant3/1 -> Logical Operator1/2
  Compare To Constant2/1 -> Logical Operator1/1
  Logical Operator1/1 -> Switch1/2
  [VBCM_OutMode_enum] -> Compare To Constant2/1, Compare To Constant3/1
  [VINP_CSWTurnSWSta_enum] -> Compare To Constant4/1, Compare To Constant5/1
  Logical Operator2/1 -> VBCM_TurnLpLActiveCmd_flg/1  "VBCM_TurnLpLActiveCmd_flg"
  Logical Operator3/1 -> VBCM_TurnLpRActiveCmd_flg/1  "VBCM_TurnLpRActiveCmd_flg"
  VINP_CSWTurnSWSta_enum/1 -> [VINP_CSWTurnSWSta_enum], Chart/4(CSW_TurnSw_Sta)
  Compare To Constant4/1 -> Logical Operator2/1
  [VPMM_PwrSta_enum] -> Compare To Constant6/1
  Compare To Constant5/1 -> Logical Operator3/2
  Compare To Constant6/1 -> Logical Operator3/1, Logical Operator2/2
  VINP_BuzzerMute_flg/1 -> Switch2/2
  Constant/1 -> Switch2/1
  Chart/5(FDC_BCM_BBuzzer_Cmd) -> Switch2/3
  Switch2/1 -> VBCM_BBuzzerCmd_flg/1  "VBCM_BBuzzerCmd_flg"

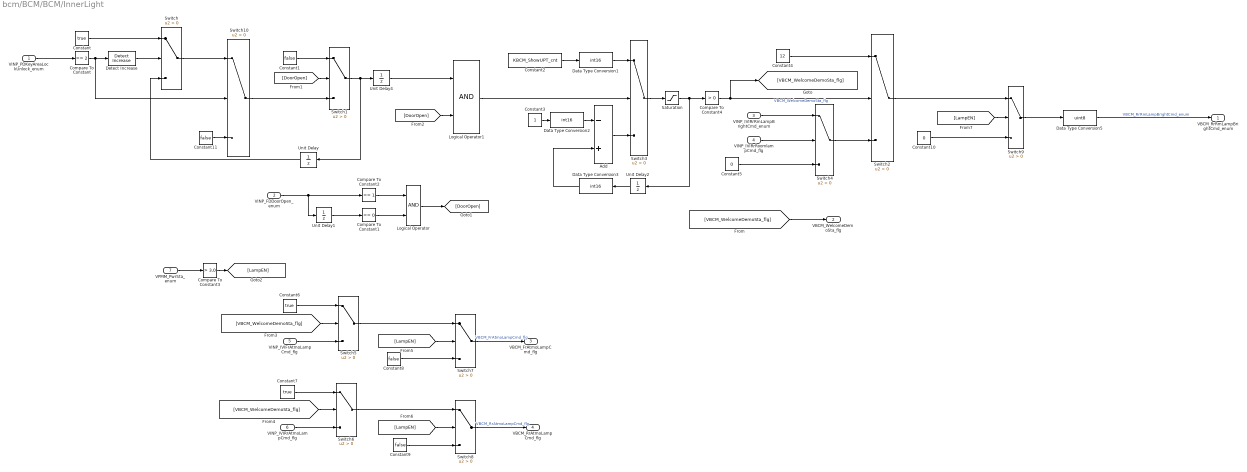
== system bcm/BCM/BCM/InnerLight ==
  VINP_PDKeyAreaLockUnlock_enum : Inport
  VINP_FDDoorOpen_enum : Inport  Port=2
  VINP_IVIRrRmLampBrightCmd_enum : Inport  Port=3
  VINP_IVIRrRoomlampCmd_flg : Inport  Port=4
  VINP_IVIFrAtmoLampCmd_flg : Inport  Port=5
  VINP_IVIRrAtmoLampCmd_flg : Inport  Port=6
  VPMM_PwrSta_enum : Inport  Port=7
  Add : Sum  Inputs=-+
  Compare To Constant : simulink/Logic and Bit Operations/Compare To Constant  relop===  const=2  OutDataTypeStr=boolean
  Compare To Constant1 : simulink/Logic and Bit Operations/Compare To Constant  relop===  const=0  OutDataTypeStr=boolean
  Compare To Constant2 : simulink/Logic and Bit Operations/Compare To Constant  relop===  const=1  OutDataTypeStr=boolean
  Compare To Constant3 : simulink/Logic and Bit Operations/Compare To Constant  relop=>  const=3.0  OutDataTypeStr=boolean
  Compare To Constant4 : simulink/Logic and Bit Operations/Compare To Constant  relop=>  const=0  OutDataTypeStr=boolean
  Constant : Constant  Value=true
  Constant{1,8..9,11} (4 alike) : Constant  Value=false
  Constant10 : Constant  Value=0
  Constant2 : Constant  Value=KBCM_ShowUPT_cnt
  Constant3 : Constant
  Constant4 : Constant  Value=12
  Constant5 : Constant  Value=0
  Constant6 : Constant  Value=true
  Constant7 : Constant  Value=true
  Data Type Conversion1 : DataTypeConversion  OutDataTypeStr=int16
  Data Type Conversion2 : DataTypeConversion  OutDataTypeStr=int16
  Data Type Conversion3 : DataTypeConversion  OutDataTypeStr=int16
  Data Type Conversion5 : DataTypeConversion  OutDataTypeStr=uint8
  Detect Increase : simulink/Logic and Bit Operations/Detect Increase  vinit=0.0  OutDataTypeStr=boolean
  Logical Operator : Logic  AllPortsSameDT=off  OutDataTypeStr=boolean
  Logical Operator1 : Logic  AllPortsSameDT=off  OutDataTypeStr=boolean
  Saturation : Saturate  UpperLimit=10000  LowerLimit=0
  Switch{,1..10} (11 alike) : Switch  Criteria=u2 > Threshold
  Unit Delay{,1..2,4} (4 alike) : UnitDelay  SampleTime=-1  HasFrameUpgradeWarning=on
  VBCM_RrRmLampBrightCmd_enum : Outport
  VBCM_WelcomeDemoSta_flg : Outport  Port=2
  VBCM_FrAtmoLampCmd_flg : Outport  Port=3
  VBCM_RrAtmoLampCmd_flg : Outport  Port=4
  wires:
  VINP_PDKeyAreaLockUnlock_enum/1 -> Compare To Constant/1
  Compare To Constant/1 -> Switch10/2, Detect Increase/1
  Constant/1 -> Switch/1
  Detect Increase/1 -> Switch/2
  Unit Delay/1 -> Switch/3
  VINP_FDDoorOpen_enum/1 -> Unit Delay1/1, Compare To Constant2/1
  Unit Delay1/1 -> Compare To Constant1/1
  Compare To Constant1/1 -> Logical Operator/2
  Compare To Constant2/1 -> Logical Operator/1
  Logical Operator/1 -> [DoorOpen]
  [DoorOpen] -> Switch1/2
  Switch10/1 -> Switch1/3
  Constant1/1 -> Switch1/1
  Unit Delay4/1 -> Logical Operator1/1
  [DoorOpen] -> Logical Operator1/2
  Saturation/1 -> Compare To Constant4/1, Unit Delay2/1
  Switch9/1 -> Data Type Conversion5/1
  Constant4/1 -> Switch2/1
  Logical Operator1/1 -> Switch3/2
  Constant2/1 -> Data Type Conversion1/1
  Data Type Conversion1/1 -> Switch3/1
  Switch3/1 -> Saturation/1
  Add/1 -> Switch3/3
  Unit Delay2/1 -> Data Type Conversion3/1
  Data Type Conversion2/1 -> Add/1
  Constant3/1 -> Data Type Conversion2/1
  VINP_IVIRrRmLampBrightCmd_enum/1 -> Switch4/1
  Compare To Constant4/1 -> [VBCM_WelcomeDemoSta_flg], Switch2/2  "VBCM_WelcomeDemoSta_flg"
  Switch4/1 -> Switch2/3
  VINP_IVIRrRoomlampCmd_flg/1 -> Switch4/2
  Constant5/1 -> Switch4/3
  Switch1/1 -> Unit Delay/1, Unit Delay4/1
  [VBCM_WelcomeDemoSta_flg] -> VBCM_WelcomeDemoSta_flg/1
  [VBCM_WelcomeDemoSta_flg] -> Switch5/2
  Switch7/1 -> VBCM_FrAtmoLampCmd_flg/1  "VBCM_FrAtmoLampCmd_flg"
  Constant6/1 -> Switch5/1
  VINP_IVIFrAtmoLampCmd_flg/1 -> Switch5/3
  Constant7/1 -> Switch6/1
  [VBCM_WelcomeDemoSta_flg] -> Switch6/2
  VINP_IVIRrAtmoLampCmd_flg/1 -> Switch6/3
  VPMM_PwrSta_enum/1 -> Compare To Constant3/1
  Compare To Constant3/1 -> [LampEN]
  [LampEN] -> Switch7/2
  Switch5/1 -> Switch7/1
  Constant8/1 -> Switch7/3
  Switch6/1 -> Switch8/1
  [LampEN] -> Switch8/2
  Constant9/1 -> Switch8/3
  Switch8/1 -> VBCM_RrAtmoLampCmd_flg/1  "VBCM_RrAtmoLampCmd_flg"
  Switch2/1 -> Switch9/1
  [LampEN] -> Switch9/2
  Constant10/1 -> Switch9/3
  Switch/1 -> Switch10/1
  Constant11/1 -> Switch10/3
  Data Type Conversion5/1 -> VBCM_RrRmLampBrightCmd_enum/1  "VBCM_RrRmLampBrightCmd_enum"
  Data Type Conversion3/1 -> Add/2

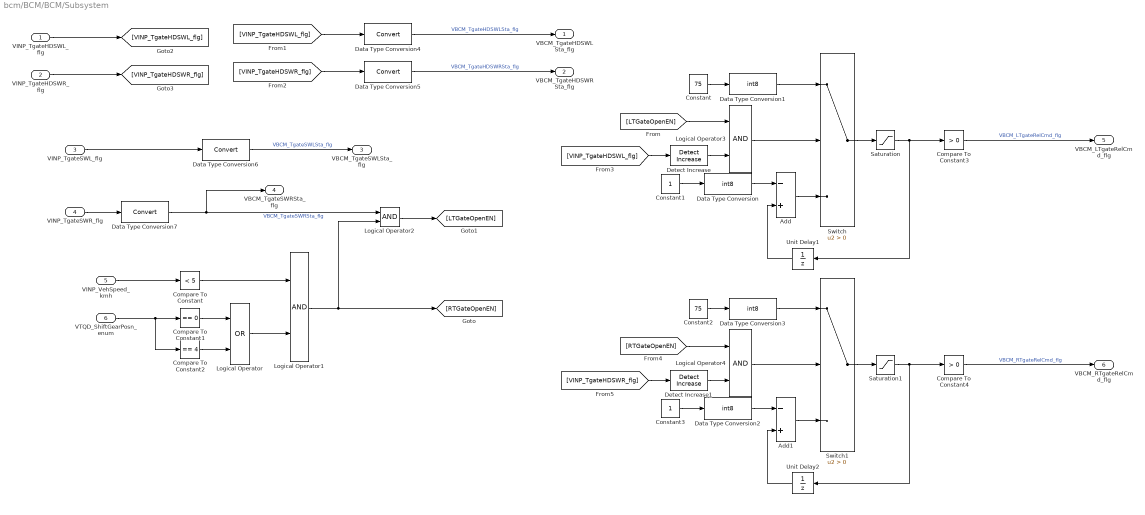
== system bcm/BCM/BCM/Subsystem ==
  VINP_TgateHDSWL_flg : Inport
  VINP_TgateHDSWR_flg : Inport  Port=2
  VINP_TgateSWL_flg : Inport  Port=3
  VINP_TgateSWR_flg : Inport  Port=4
  VINP_VehSpeed_kmh : Inport  Port=5
  VTQD_ShiftGearPosn_enum : Inport  Port=6
  Add : Sum  Inputs=-+
  Add1 : Sum  Inputs=-+
  Compare To Constant : simulink/Logic and Bit Operations/Compare To Constant  relop=<  const=5  OutDataTypeStr=boolean
  Compare To Constant1 : simulink/Logic and Bit Operations/Compare To Constant  relop===  const=0  OutDataTypeStr=boolean
  Compare To Constant2 : simulink/Logic and Bit Operations/Compare To Constant  relop===  const=4  OutDataTypeStr=boolean
  Compare To Constant3 : simulink/Logic and Bit Operations/Compare To Constant  relop=>  const=0  OutDataTypeStr=boolean
  Compare To Constant4 : simulink/Logic and Bit Operations/Compare To Constant  relop=>  const=0  OutDataTypeStr=boolean
  Constant : Constant  Value=75
  Constant1 : Constant
  Constant2 : Constant  Value=75
  Constant3 : Constant
  Data Type Conversion{,1..3} (4 alike) : DataTypeConversion  OutDataTypeStr=int8
  Data Type Conversion{4..7} (4 alike) : DataTypeConversion
  Detect Increase : simulink/Logic and Bit Operations/Detect Increase  vinit=0.0  OutDataTypeStr=boolean
  Detect Increase1 : simulink/Logic and Bit Operations/Detect Increase  vinit=0.0  OutDataTypeStr=boolean
  Logical Operator : Logic  Operator=OR  AllPortsSameDT=off  OutDataTypeStr=boolean
  Logical Operator{1..4} (4 alike) : Logic  AllPortsSameDT=off  OutDataTypeStr=boolean
  Saturation : Saturate  UpperLimit=75  LowerLimit=0
  Saturation1 : Saturate  UpperLimit=75  LowerLimit=0
  Switch : Switch  Criteria=u2 > Threshold
  Switch1 : Switch  Criteria=u2 > Threshold
  Unit Delay1 : UnitDelay  SampleTime=-1  HasFrameUpgradeWarning=on
  Unit Delay2 : UnitDelay  SampleTime=-1  HasFrameUpgradeWarning=on
  VBCM_TgateHDSWLSta_flg : Outport
  VBCM_TgateHDSWRSta_flg : Outport  Port=2
  VBCM_TgateSWLSta_flg : Outport  Port=3
  VBCM_TgateSWRSta_flg : Outport  Port=4
  VBCM_LTgateRelCmd_flg : Outport  Port=5
  VBCM_RTgateRelCmd_flg : Outport  Port=6
  wires:
  VINP_VehSpeed_kmh/1 -> Compare To Constant/1
  VTQD_ShiftGearPosn_enum/1 -> Compare To Constant2/1, Compare To Constant1/1
  Compare To Constant1/1 -> Logical Operator/1
  Compare To Constant2/1 -> Logical Operator/2
  Logical Operator/1 -> Logical Operator1/2
  Compare To Constant/1 -> Logical Operator1/1
  Logical Operator1/1 -> Logical Operator2/2, [RTGateOpenEN]
  VINP_TgateSWR_flg/1 -> Data Type Conversion7/1
  Logical Operator2/1 -> [LTGateOpenEN]
  VINP_TgateSWL_flg/1 -> Data Type Conversion6/1
  VINP_TgateHDSWL_flg/1 -> [VINP_TgateHDSWL_flg]
  VINP_TgateHDSWR_flg/1 -> [VINP_TgateHDSWR_flg]
  [VINP_TgateHDSWL_flg] -> Data Type Conversion4/1
  Data Type Conversion5/1 -> VBCM_TgateHDSWRSta_flg/1  "VBCM_TgateHDSWRSta_flg"
  Logical Operator3/1 -> Switch/2
  [LTGateOpenEN] -> Logical Operator3/1
  Detect Increase/1 -> Logical Operator3/2
  [VINP_TgateHDSWL_flg] -> Detect Increase/1
  Constant/1 -> Data Type Conversion1/1
  Switch/1 -> Saturation/1
  Add/1 -> Switch/3
  Unit Delay1/1 -> Add/2
  Saturation/1 -> Compare To Constant3/1, Unit Delay1/1
  Constant1/1 -> Data Type Conversion/1
  Data Type Conversion/1 -> Add/1
  Data Type Conversion1/1 -> Switch/1
  Compare To Constant3/1 -> VBCM_LTgateRelCmd_flg/1  "VBCM_LTgateRelCmd_flg"
  Compare To Constant4/1 -> VBCM_RTgateRelCmd_flg/1  "VBCM_RTgateRelCmd_flg"
  Data Type Conversion3/1 -> Switch1/1
  Data Type Conversion2/1 -> Add1/1
  Constant3/1 -> Data Type Conversion2/1
  Saturation1/1 -> Unit Delay2/1, Compare To Constant4/1
  Unit Delay2/1 -> Add1/2
  Add1/1 -> Switch1/3
  Switch1/1 -> Saturation1/1
  Constant2/1 -> Data Type Conversion3/1
  [VINP_TgateHDSWR_flg] -> Detect Increase1/1
  Detect Increase1/1 -> Logical Operator4/2
  [RTGateOpenEN] -> Logical Operator4/1
  Logical Operator4/1 -> Switch1/2
  Data Type Conversion4/1 -> VBCM_TgateHDSWLSta_flg/1  "VBCM_TgateHDSWLSta_flg"
  [VINP_TgateHDSWR_flg] -> Data Type Conversion5/1
  Data Type Conversion6/1 -> VBCM_TgateSWLSta_flg/1  "VBCM_TgateSWLSta_flg"
  Data Type Conversion7/1 -> VBCM_TgateSWRSta_flg/1, Logical Operator2/1  "VBCM_TgateSWRSta_flg"

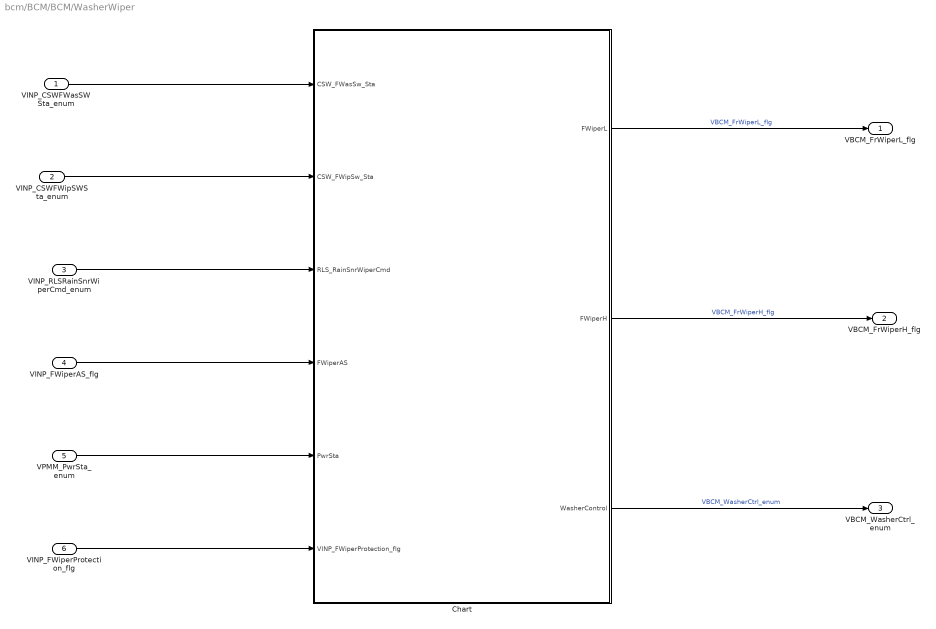
== system bcm/BCM/BCM/WasherWiper ==
  VINP_CSWFWasSWSta_enum : Inport
  VINP_CSWFWipSWSta_enum : Inport  Port=2
  VINP_RLSRainSnrWiperCmd_enum : Inport  Port=3
  VINP_FWiperAS_flg : Inport  Port=4
  VPMM_PwrSta_enum : Inport  Port=5
  VINP_FWiperProtection_flg : Inport  Port=6
  Chart : Stateflow chart  TreatAsAtomicUnit=on
  VBCM_FrWiperL_flg : Outport
  VBCM_FrWiperH_flg : Outport  Port=2
  VBCM_WasherCtrl_enum : Outport  Port=3
  wires:
  VINP_FWiperProtection_flg/1 -> Chart/6(VINP_FWiperProtection_flg)
  Chart/1(FWiperL) -> VBCM_FrWiperL_flg/1  "VBCM_FrWiperL_flg"
  Chart/2(FWiperH) -> VBCM_FrWiperH_flg/1  "VBCM_FrWiperH_flg"
  VINP_FWiperAS_flg/1 -> Chart/4(FWiperAS)
  VINP_CSWFWipSWSta_enum/1 -> Chart/2(CSW_FWipSw_Sta)
  VPMM_PwrSta_enum/1 -> Chart/5(PwrSta)
  VINP_CSWFWasSWSta_enum/1 -> Chart/1(CSW_FWasSw_Sta)
  VINP_RLSRainSnrWiperCmd_enum/1 -> Chart/3(RLS_RainSnrWiperCmd)
  Chart/3(WasherControl) -> VBCM_WasherCtrl_enum/1  "VBCM_WasherCtrl_enum"

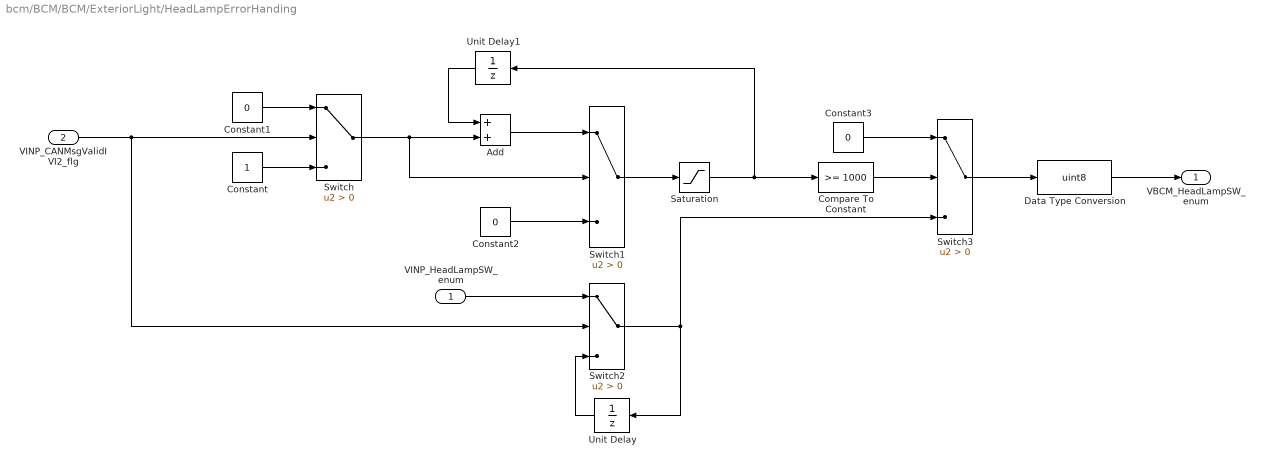
== system bcm/BCM/BCM/ExteriorLight/HeadLampErrorHanding ==
  VINP_HeadLampSW_enum : Inport
  VINP_CANMsgValidIVI2_flg : Inport  Port=2
  Add : Sum
  Compare To Constant : simulink/Logic and Bit Operations/Compare To Constant  relop=>=  const=1000  OutDataTypeStr=boolean
  Constant : Constant
  Constant1 : Constant  Value=0
  Constant2 : Constant  Value=0
  Constant3 : Constant  Value=0
  Data Type Conversion : DataTypeConversion  OutDataTypeStr=uint8
  Saturation : Saturate  UpperLimit=1000  LowerLimit=0
  Switch{,1..3} (4 alike) : Switch  Criteria=u2 > Threshold
  Unit Delay : UnitDelay  SampleTime=-1  HasFrameUpgradeWarning=on
  Unit Delay1 : UnitDelay  SampleTime=-1  HasFrameUpgradeWarning=on
  VBCM_HeadLampSW_enum : Outport
  wires:
  VINP_CANMsgValidIVI2_flg/1 -> Switch2/2, Switch/2
  Switch2/1 -> Switch3/3, Unit Delay/1
  Unit Delay/1 -> Switch2/3
  VINP_HeadLampSW_enum/1 -> Switch2/1
  Switch/1 -> Switch1/2, Add/2
  Unit Delay1/1 -> Add/1
  Add/1 -> Switch1/1
  Constant/1 -> Switch/3
  Constant1/1 -> Switch/1
  Constant2/1 -> Switch1/3
  Constant3/1 -> Switch3/1
  Switch3/1 -> Data Type Conversion/1
  Compare To Constant/1 -> Switch3/2
  Saturation/1 -> Unit Delay1/1, Compare To Constant/1
  Switch1/1 -> Saturation/1
  Data Type Conversion/1 -> VBCM_HeadLampSW_enum/1
